simulink model "TestModel"  (Simulink 8.5)
settings: Solver=VariableStepDiscrete  StartTime=0.0  StopTime=1000  RelTol=1e-3
settings Model: Creator=tsprock3  LastModifiedBy=tsprock3
settings DebuggingCC: SolverPrmCheckMsg=warning  FcnCallInpInsideContextMsg=EnableAllAsWarning  SimStateOlderReleaseMsg=warning
settings GRTTargetCC: CombineOutputUpdateFcns=on  GRTInterface=off

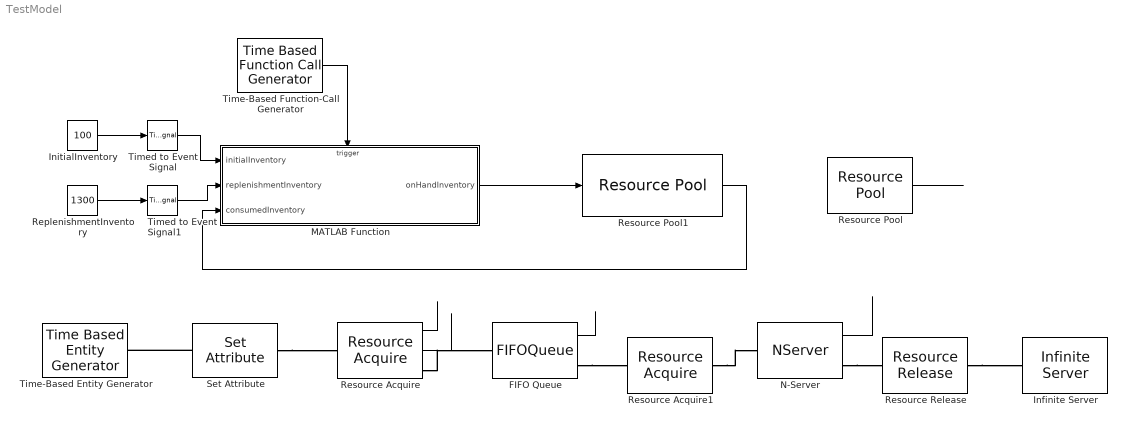
== system TestModel ==
  FIFO Queue : FIFOQueue  StatNumberDeparted=on
  Infinite Server : InfiniteServer  ServiceTime=inf
  InitialInventory : Constant  Value=100
  MATLAB Function : MATLAB Function  TreatAsAtomicUnit=on
  N-Server : NServer  ServiceTime=3.5  StatNumberDeparted=on
  ReplenishmentInventory : Constant  Value=1300
  Resource Acquire : ResourceAcquire  ResourceName=rawMaterial  ResourceAmountSource=Attribute  ResourceAmount=rawMaterialQty  Capacity=100  StatNumberDeparted=on  StatNumberInBlock=on  EvaluatedResourceAmount={ []}
      settings: OutputPortMap=o0,o1
  Resource Acquire1 : ResourceAcquire  ResourceName=Operator  ResourceAmountSource=Attribute  ResourceAmount=operatorCount  EvaluatedResourceAmount={ []}
  Resource Pool : ResourcePool  ResourceName=Operator  ResourceAmount=1000  StatAmountInUse=on
  Resource Pool1 : ResourcePool  ResourceName=rawMaterial  ResourceAmountSource=Signal port  ResourceAmount=100  StatAmountInUse=on
  Resource Release : ResourceRelease  ResourceReleaseAction=Selected  ResourceName=Operator
  Set Attribute : SetAttribute  AttributeName=operatorCount|rawMaterialQty  AttributeFrom=Dialog|Dialog  AttributeValue=1|4  AttributeTreatAsVector=1|1  EvaluatedAttributeValue={ 1;4}
  Time-Based Entity Generator : TimeBasedEntityGenerator  Period=3
  Time-Based Function-Call Generator : TimeBasedFunctionCallGenerator
  Timed to Event Signal : TimedToEventSignal
  Timed to Event Signal1 : TimedToEventSignal
  wires:
  Resource Pool/1 -> ?
  InitialInventory/1 -> Timed to Event Signal/1
  Timed to Event Signal/1 -> MATLAB Function/1(initialInventory)
  Resource Acquire/2 -> ?
  Resource Acquire/1 -> ?
  FIFO Queue/1 -> ?
  N-Server/1 -> ?
  ReplenishmentInventory/1 -> Timed to Event Signal1/1
  Timed to Event Signal1/1 -> MATLAB Function/2(replenishmentInventory)
  MATLAB Function/1(onHandInventory) -> Resource Pool1/1
  Time-Based Function-Call Generator/1 -> MATLAB Function/Trigger
  Resource Pool1/1 -> MATLAB Function/3(consumedInventory)
  connections:
  Resource Acquire/RConn1 -- FIFO Queue/LConn1
  Set Attribute/LConn1 -- Time-Based Entity Generator/RConn1
  Set Attribute/RConn1 -- Resource Acquire/LConn1
  FIFO Queue/RConn1 -- Resource Acquire1/LConn1
  Resource Acquire1/RConn1 -- N-Server/LConn1
  N-Server/RConn1 -- Resource Release/LConn1
  Resource Release/RConn1 -- Infinite Server/LConn1

== matlab function MATLAB Function ==
  data: initialInventory input double; onHandInventory output double; replenishmentInventory input double; consumedInventory input double
  events: trigger input FUNCTION_CALL_EVENT
function onHandInventory = fcn(initialInventory ,replenishmentInventory, consumedInventory)
%#codegen

coder.extrinsic('num2str', 'set_param')

onHandInventory = initialInventory+replenishmentInventory;

if consumedInventory > onHandInventory-25
    set_param('TestModel/ReplenishmentInventory','Value',num2str(replenishmentInventory+100));
end
